simulink model "AEB_Model"  (R2025b)
settings: Solver=FixedStepDiscrete  StartTime=0.0  StopTime=1  FixedStep=0.01  RelTol=1e-3
settings Model: Creator=pipat  LastModifiedBy=pipat
settings OptimizationCC: DefaultParameterBehavior=Inlined  EnhancedBackFolding=on  PassReuseOutputArgsAs=Individual arguments  ZeroExternalMemoryAtStartup=off  ZeroInternalMemoryAtStartup=off  OptimizeBlockOrder=speed  DifferentSizesBufferReuse=on  OptimizationCustomize=off  EfficientTunableParamExpr=on
settings DebuggingCC: ParameterTunabilityLossMsg=error
settings SFSimCC: MATLABDynamicMemAlloc=off
settings RTWCC: SystemTargetFile=ert.tlc  TemplateMakefile=ert_default_tmf  GenerateReport=on  Description=Embedded Coder
settings CodeAppCC: ForceParamTrailComments=on  IgnoreCustomStorageClasses=off  OperatorAnnotations=on  SimulinkDataObjDesc=on  SFDataObjDesc=on  InsertBlockDesc=on
settings ERTTargetCC: ERTCustomFileTemplate=example_file_process.tlc  TargetLangStandard=C99 (ISO)  GenerateSampleERTMain=on

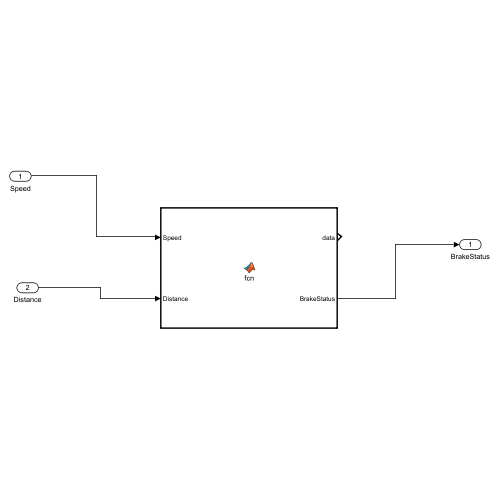
[thumbnail: Simulink's stored preview of the top-level diagram]
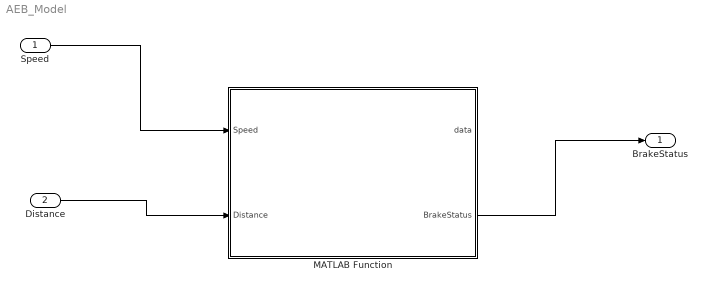
== system AEB_Model ==
  Speed : Inport  PortDimensions=1
  Distance : Inport  Port=2  PortDimensions=1
  MATLAB Function : MATLAB Function  TreatAsAtomicUnit=on
  BrakeStatus : Outport  PortDimensions=1
  wires:
  Speed/1 -> MATLAB Function/1(Speed)
  Distance/1 -> MATLAB Function/2(Distance)
  MATLAB Function/2(BrakeStatus) -> BrakeStatus/1

== matlab function AEB_Model/MATLAB Function ==
  data: data output; Speed input; BrakeStatus output; Distance input
function [data, BrakeStatus]= fcn(Speed, Distance)
    if Distance < 10 && Speed > 0
        BrakeStatus = 1;      % Full brake
    elseif Distance < 20
        BrakeStatus = 0.5;    % Partial brake
    else
        BrakeStatus = 0;      % No brake
    end
end
